simulink model "Exp2_19EE10039_Mansi_PartA"  (R2021a)
settings: Solver=VariableStepAuto  StartTime=0.0  StopTime=0.005  RelTol=1e-3
libraries: spsCurrentMeasurementLib x3, spsVoltageMeasurementLib x3, spsSeriesRLCBranchLib x2, spsDCVoltageSourceLib x1, spsDiodeLib x1, spsLinearTransformerLib x1, spsMosfetLib x1, spsMultimeterLib x1, spspowerguiLib x1
settings Model: Creator=mansi  LastModifiedBy=mansi

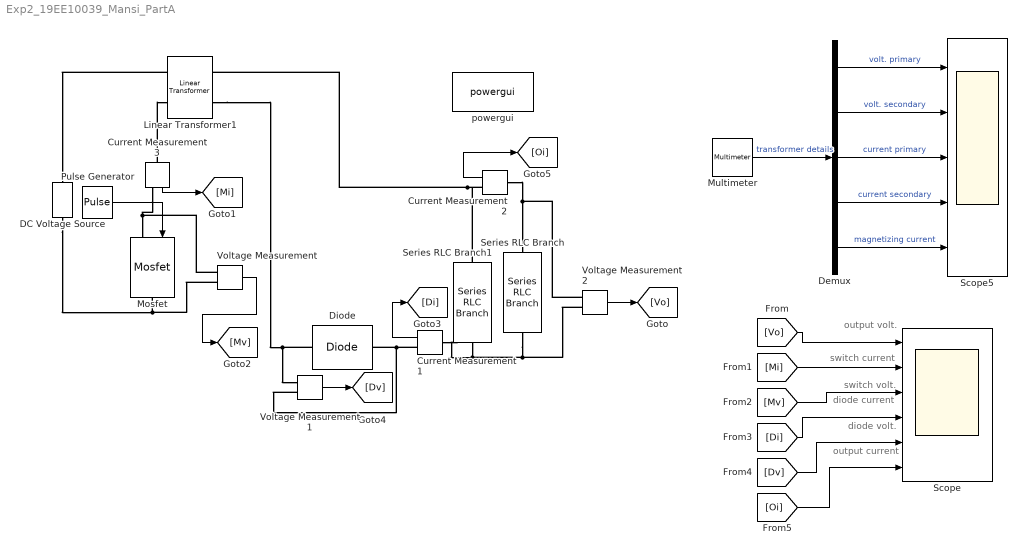
== system Exp2_19EE10039_Mansi_PartA ==
  note: switch current
  note: switch volt.
  note: diode volt.
  note: diode current
  note: output volt.
  note: output current
  Current Measurement1 : spsCurrentMeasurementLib/Current Measurement  PhasorSimulation=off  OutputType=Complex  PSBequivalent=0
  Current Measurement2 : spsCurrentMeasurementLib/Current Measurement  PhasorSimulation=off  OutputType=Complex  PSBequivalent=0
  Current Measurement3 : spsCurrentMeasurementLib/Current Measurement  PhasorSimulation=off  OutputType=Complex  PSBequivalent=0
  DC Voltage Source : spsDCVoltageSourceLib/DC Voltage Source  Amplitude=20  Measurements=None
  Demux : Demux  Outputs=5
  Diode : spsDiodeLib/Diode  Ron=1e-6  Lon=0  Vf=0  IC=0  UseSnubber=0  Rs=1e12  Cs=0  Measurements=off
  Linear Transformer1 : spsLinearTransformerLib/Linear Transformer  UNITS=SI  NominalPower=[20 100000 ]  winding1=[30 0 0]  winding2=[10 0 0]  ThreeWindings=off  winding3=[3.15e+05 0.7938 0.084225]  RmLm=[inf 250e-6]  Measurements=All voltages and currents  DataType=on
  Mosfet : spsMosfetLib/Mosfet  Ron=1e-6  Lon=0  Rd=1e-6  Vfd=0  IC=0  Rs=1e12  Cs=inf  Measurements=off
  Multimeter : spsMultimeterLib/Multimeter  PhasorSimulation=off  OutputType=Complex  sel=[1 2 3 4 6]  L=7  Gain=[1 1 1 1 1]  yselected={'Uw1: Linear Transformer1','Uw2: Linear Transformer1','Iw1: Linear Transformer1','Iw2: Linear Transformer1','Imag: Linear Transformer1'};  PSBOutputType=1  PSBequivalent=0  AxesSetting=[0,0.1,-100,100]  Display=0  SavedBlockNames=-11
  Pulse Generator : DiscretePulseGenerator  PulseType=Time based  Period=1/100000  PulseWidth=50
  Scope : Scope  NumInputPorts=6
  Scope5 : Scope  NumInputPorts=5
  Series RLC Branch : spsSeriesRLCBranchLib/Series RLC Branch  LConnTagsString=__new0  RConnTagsString=__new0  BranchType=R  Resistance=1.5  Inductance=1e-3  SetiL0=off  InitialCurrent=0  Capacitance=1e-6  Setx0=off  InitialVoltage=0  Measurements=None
  Series RLC Branch1 : spsSeriesRLCBranchLib/Series RLC Branch  LConnTagsString=__new0  RConnTagsString=__new0  BranchType=C  Resistance=1  Inductance=1e-3  SetiL0=off  InitialCurrent=0  Capacitance=100e-6  Setx0=off  InitialVoltage=0  Measurements=None
  Voltage Measurement : spsVoltageMeasurementLib/Voltage Measurement  PhasorSimulation=off  OutputType=Complex  PSBequivalent=0
  Voltage Measurement1 : spsVoltageMeasurementLib/Voltage Measurement  PhasorSimulation=off  OutputType=Complex  PSBequivalent=0
  Voltage Measurement2 : spsVoltageMeasurementLib/Voltage Measurement  PhasorSimulation=off  OutputType=Complex  PSBequivalent=0
  powergui : spspowerguiLib/powergui  Priority=1  SimulationMode=Discrete  SampleTime=1e-7  frequency=60  Iterations=50  frequencyindice=0  Pbase=100e6  ErrMax=1e-4  UnitsV=kV  UnitsW=MW  buscounter=0  FunctionMessages=off  echomessages=off  EnableUseOfTLC=off  CurrentSourceSwitches=off  DisableSnubberDevices=off  DisableRonSwitches=off  DisableVfSwitches=off  DisplayEquations=off  AutomaticDiscreteSolvers=off  SolverType=Tustin/Backward Euler (TBE)  Interpol=off  ExternalGateDelay=off  methode=off  Ts=100  x0status=blocks  SPID=on  SwTol=0  HookPort=off  NonlinearTolerance=1e-4  nMaxIteration=100  ContinueOnMaxIteration=off  RestoreLinks=warning  ResistiveCurrentMeasurement=off  Frange=[0:2:500]  Ylog=off  Xlog=on  ShowGrid=off  save=off  variable=ZData  structure=0  ZoomFFT=off  StartTime=0.0  cycles=1  DisplayStyle=1  fundamental=60  FreqAxis=off  MaxFrequency=1000  frequencyindicesteady=1  RmsSteady=1  display=off
  wires:
  Voltage Measurement2/1 -> [Vo]
  Voltage Measurement/1 -> [Mv]
  Voltage Measurement1/1 -> [Dv]
  [Vo] -> Scope/1
  [Mi] -> Scope/2
  [Mv] -> Scope/3
  [Di] -> Scope/4
  [Dv] -> Scope/5
  Pulse Generator/1 -> Mosfet/1
  Current Measurement3/1 -> [Mi]
  Current Measurement2/1 -> [Oi]
  [Oi] -> Scope/6
  Demux/1 -> Scope5/1  "volt. primary"
  Demux/3 -> Scope5/3  "current primary"
  Demux/5 -> Scope5/5  "magnetizing current"
  Demux/2 -> Scope5/2  "volt. secondary"
  Demux/4 -> Scope5/4  "current secondary"
  Multimeter/1 -> Demux/1  "transformer details"
  Current Measurement1/1 -> [Di]
  connections:
  Linear Transformer1/LConn1 -- DC Voltage Source/RConn1
  Voltage Measurement/LConn2 -- DC Voltage Source/LConn1 -- Mosfet/RConn1
  Diode/LConn1 -- Voltage Measurement1/LConn1 -- Linear Transformer1/RConn2
  Voltage Measurement1/LConn2 -- Current Measurement1/RConn1 -- Diode/RConn1
  Current Measurement2/LConn1 -- Voltage Measurement2/LConn2 -- Series RLC Branch/LConn1
  Current Measurement3/LConn1 -- Linear Transformer1/LConn2
  Current Measurement3/RConn1 -- Voltage Measurement/LConn1 -- Mosfet/LConn1
  Series RLC Branch1/LConn1 -- Current Measurement2/RConn1 -- Linear Transformer1/RConn1
  Series RLC Branch/RConn1 -- Voltage Measurement2/LConn1 -- Series RLC Branch1/RConn1 -- Current Measurement1/LConn1
